simulink model "balanceLQRhostTest"  (Simulink 8.1)
settings: Solver=ode3  StartTime=0.0  StopTime=inf  RelTol=1e-3
StopFcn:
  | subplot(3,1,1);
  | plot(Data.time,Data.signals(1,1).values,'-r','LineWidth',1.5)
  | legend('Angle');
  | grid;
  | ylabel('alpha [deg]');
  | title('Pendulum');
  | subplot(3,1,2);
  | plot(Data.time,Data.signals(1,4).values,'-r','LineWidth',1.5)
  | hold on;
  | plot(Data.time,Data.signals(1,3).values,'-b','LineWidth',1.5)
  | grid;
  | legend('theta','setvalue');
  | ylabel('Arm [deg]');
  | subplot(3,1,3);
  | plot(Data.time,Data.signals(1,5).values,'-r','LineWidth',0.5)
  | legend('V');
  | grid;
  | ylabel('Voltage [V]');
libraries: aerolibconvert2 x5
settings Model: Creator=ThanhNhan  LastModifiedBy=ThanhNhan
settings DataIOCC: SignalLoggingSaveFormat=Dataset
settings OptimizationCC: ExpressionDepthLimit=128  OptimizeModelRefInitCode=on  LifeSpan=Inf
settings DebuggingCC: FcnCallInpInsideContextMsg=EnableAllAsError
settings RTWCC: SystemTargetFile=stm32f4.tlc  TemplateMakefile=ert_default_tmf  Description=STM32F4 Target  ProcessScript=stm32f4_make_rtw_hook
settings CodeAppCC: IgnoreCustomStorageClasses=off
settings STFCustomTargetCC: CodeReplacementLibrary=ANSI_C  GenerateSampleERTMain=on  ModelReferenceCompliant=off  CombineOutputUpdateFcns=on  ERTCustomFileBanners=on  SupportContinuousTime=off  SupportNonInlinedSFcns=off  MATLABClassNameForMDSCustomization=Simulink.SoftwareTarget.ERTCustomization  GRTInterface=off  SystemTargetFile=stm32f4.tlc
settings ERTTargetCC: CodeReplacementLibrary=ANSI_C  MultiwordLength=2048  GenerateSampleERTMain=on  ModelReferenceCompliant=off  ParMdlRefBuildCompliant=off  CompOptLevelCompliant=off  ConcurrentExecutionCompliant=off  ERTFirstTimeCompliant=off  ModelStepFunctionPrototypeControlCompliant=off  CPPClassGenCompliant=off  InlinedParameterPlacement=NonHierarchical  ERTCustomFileTemplate=example_file_process.tlc  ConvertIfToSwitch=off  SuppressUnreachableDefaultCases=off

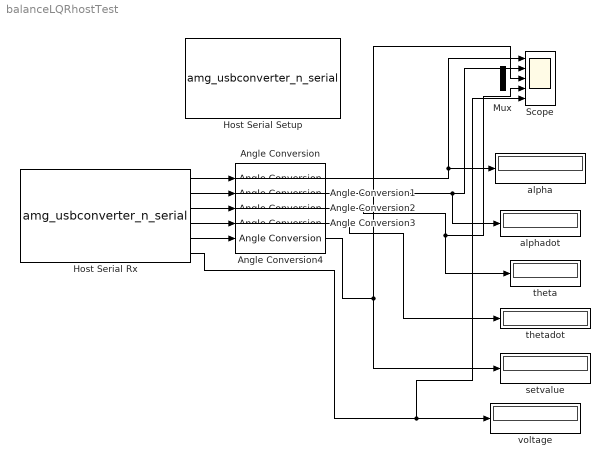
== system balanceLQRhostTest ==
  Angle Conversion{,1..4} (5 alike) : aerolibconvert2/Angle Conversion  IU=rad  OU=deg
  Host Serial Rx : S-Function  Priority=1  FunctionName=amg_usbconverter_n_serial  Parameters=configuration,port,transfer,baudrate,stopbit,inputtype,outputtype,binheaderarray,binterminatorarray,asciiheader,asciiterminator,bindatalength,packetmode,timeout,sampletime,sampletimestr,blockid  EnableBusSupport=off  mask(amg_usbconverter_n_serial){configuration=Rx, port=COM4, baudrate=115200, databits=8, parity=None, stopbit=1, flowcontrol=None, advanceoptions=off, rxbuffersize=2048, txbuffersize=2048, transfer=Blocking, timeout=5, packetmode=Binary, binheader='7E 7E', binterminator='03 03', porttype_double=6, porttype_single=0, porttype_int8=0, porttype_uint8=0, porttype_int16=0, porttype_uint16=0, porttype_int32=0, porttype_uint32=0, asciiformat='%d,%f', rx_asciiterminator=LF (0x0A - "\n"), tx_asciiterminator=LF (0x0A - "\n"), inputtype=[0], outputtype=[6  0 0 0 0 0 0], binheaderarray=[2 126  126], binterminatorarray=[2 3  3], bindatalength=48, asciiheader=['%d,%f' uint8(10)], asciiterminator=[1 10], sampletime=0.01, sampletimestr=0.01, blockid=HostSerialRx}
      mask prompts: baudrate "Baud rate (bps)"; databits "Data bits"; stopbit "Stop bit"; flowcontrol "Hardware flow control"; advanceoptions "Advance options"; rxbuffersize "Rx buffer size (bytes)"; txbuffersize "Tx buffer size (bytes)"; timeout "Wait time-out (Seconds)"; packetmode "Packet mode"; binheader "Binary header (example: '7E 7E')"; binterminator "Binary terminator (example: '03 03')"; porttype_double "Number of data port, type DOUBLE"; porttype_single "Number of data port, type SINGLE"; porttype_int8 "Number of data port, type INT8"; porttype_uint8 "Number of data port, type UINT8"; porttype_int16 "Number of data port, type INT16"; porttype_uint16 "Number of data port, type UINT16"; porttype_int32 "Number of data port, type INT32"; porttype_uint32 "Number of data port, type UINT32"; asciiformat "Ascii format"; rx_asciiterminator "End of packet"; tx_asciiterminator "End of packet"; inputtype "Input data type"; outputtype "Output data type"; binheaderarray "Binary header"; binterminatorarray "Binary terminator"; bindatalength "Binary data length"; asciiheader "Ascii header (printf format)"; asciiterminator "Ascii terminator"; sampletime "Sample time (sec)"; sampletimestr "Compiled sample time (sec) in string"
      mask init:
      | amg_usbconverter_n_serial_callback('init');
      mask Help: web(fullfile(waijungdocroot,'amg_usbconverter_n_uart.htm'), '-browser')
      mask TypeOptions configuration: Setup | Tx | Rx
      mask Callback configuration: amg_usbconverter_n_serial_callback('configuration');
      mask TypeOptions port: COM1 | COM2 | COM4
      mask Callback port: amg_usbconverter_n_serial_callback('port');
      mask Callback baudrate: amg_usbconverter_n_serial_callback('baudrate');
      mask TypeOptions databits: 8
      mask TypeOptions parity: None
      mask TypeOptions stopbit: 1 | 1.5 | 2
      mask TypeOptions flowcontrol: None | RTS | CTS | RTS/CTS
      mask Callback flowcontrol: amg_usbconverter_n_serial_callback('flowcontrol');
      mask Callback advanceoptions: amg_usbconverter_n_serial_callback('advanceoptions');
      mask TypeOptions rxbuffersize: 16 | 32 | 64 | 128 | 256 | 512 | 1024 | 2048
      mask TypeOptions txbuffersize: 16 | 32 | 64 | 128 | 256 | 512 | 1024 | 2048
      mask TypeOptions transfer: Blocking | Non-Blocking
      mask Callback transfer: amg_usbconverter_n_serial_callback('transfer');
      mask TypeOptions packetmode: Ascii | Binary
      mask Callback packetmode: amg_usbconverter_n_serial_callback('packetmode');
      mask Callback binheader: amg_usbconverter_n_serial_callback('binheader');
      mask Callback binterminator: amg_usbconverter_n_serial_callback('binterminator');
      mask Callback porttype_double: amg_usbconverter_n_serial_callback('porttype');
      mask Callback porttype_single: amg_usbconverter_n_serial_callback('porttype');
      mask Callback porttype_int8: amg_usbconverter_n_serial_callback('porttype');
      mask Callback porttype_uint8: amg_usbconverter_n_serial_callback('porttype');
      mask Callback porttype_int16: amg_usbconverter_n_serial_callback('porttype');
      mask Callback porttype_uint16: amg_usbconverter_n_serial_callback('porttype');
      mask Callback porttype_int32: amg_usbconverter_n_serial_callback('porttype');
      mask Callback porttype_uint32: amg_usbconverter_n_serial_callback('porttype');
      mask Callback asciiformat: amg_usbconverter_n_serial_callback('asciiformat');
      mask TypeOptions rx_asciiterminator: CR (0x0D - "\r") | LF (0x0A - "\n") | CRLF (0x0D 0x0A - "\r\n")
      mask Callback rx_asciiterminator: amg_usbconverter_n_serial_callback('rx_asciiterminator');
      mask TypeOptions tx_asciiterminator: CR (0x0D - "\r") | LF (0x0A - "\n") | CRLF (0x0D 0x0A - "\r\n") | None
      mask Callback tx_asciiterminator: amg_usbconverter_n_serial_callback('tx_asciiterminator');
      mask Callback sampletime: amg_usbconverter_n_serial_callback('sampletime');
      mask Callback sampletimestr: amg_usbconverter_n_serial_callback('sampletimestr');
      mask Callback blockid: amg_usbconverter_n_serial_callback('blockid');
      mask Display: text(0.05, 0.5, 'Port: COM4\nPacket: Binary\nTransfer: Blocking\nTs (sec): 0.01','ver','middle','hor','left');port_label('output', 1,'double');port_label('output', 2,'double');port_label('output', 3,'double');port_label('output', 4,'double');port_label('output', 5,'double');port_label('output', 6,'double');
  Host Serial Setup : S-Function  Priority=1  FunctionName=amg_usbconverter_n_serial  Parameters=configuration,port,transfer,baudrate,stopbit,inputtype,outputtype,binheaderarray,binterminatorarray,asciiheader,asciiterminator,bindatalength,packetmode,timeout,sampletime,sampletimestr,blockid  EnableBusSupport=off  mask(amg_usbconverter_n_serial){configuration=Setup, port=COM4, baudrate=115200, databits=8, parity=None, stopbit=1, flowcontrol=None, advanceoptions=off, rxbuffersize=2048, txbuffersize=2048, transfer=Blocking, timeout=5, packetmode=Binary, binheader='7E 7E', binterminator='03 03', porttype_double=1, porttype_single=0, porttype_int8=1, porttype_uint8=0, porttype_int16=0, porttype_uint16=0, porttype_int32=0, porttype_uint32=0, asciiformat='%d,%f', rx_asciiterminator=CRLF (0x0D 0x0A - "\r\n"), tx_asciiterminator=CR (0x0D - "\r"), inputtype=[0], outputtype=[0], binheaderarray=[2 126  126], binterminatorarray=[2 3  3], bindatalength=0, asciiheader='', asciiterminator=[0], sampletime=inf, sampletimestr=0.01, blockid=HostSerialSetup}
      mask prompts: baudrate "Baud rate (bps)"; databits "Data bits"; stopbit "Stop bit"; flowcontrol "Hardware flow control"; advanceoptions "Advance options"; rxbuffersize "Rx buffer size (bytes)"; txbuffersize "Tx buffer size (bytes)"; timeout "Wait time-out (Seconds)"; packetmode "Packet mode"; binheader "Binary header (example: '7E 7E')"; binterminator "Binary terminator (example: '03 03')"; porttype_double "Number of data port, type DOUBLE"; porttype_single "Number of data port, type SINGLE"; porttype_int8 "Number of data port, type INT8"; porttype_uint8 "Number of data port, type UINT8"; porttype_int16 "Number of data port, type INT16"; porttype_uint16 "Number of data port, type UINT16"; porttype_int32 "Number of data port, type INT32"; porttype_uint32 "Number of data port, type UINT32"; asciiformat "Ascii format"; rx_asciiterminator "End of packet"; tx_asciiterminator "End of packet"; inputtype "Input data type"; outputtype "Output data type"; binheaderarray "Binary header"; binterminatorarray "Binary terminator"; bindatalength "Binary data length"; asciiheader "Ascii header (printf format)"; asciiterminator "Ascii terminator"; sampletime "Sample time (sec)"; sampletimestr "Compiled sample time (sec) in string"
      mask init:
      | amg_usbconverter_n_serial_callback('init');
      mask Help: web(fullfile(waijungdocroot,'amg_usbconverter_n_uart.htm'), '-browser')
      mask TypeOptions configuration: Setup | Tx | Rx
      mask Callback configuration: amg_usbconverter_n_serial_callback('configuration');
      mask TypeOptions port: COM1 | COM2 | COM4
      mask Callback port: amg_usbconverter_n_serial_callback('port');
      mask Callback baudrate: amg_usbconverter_n_serial_callback('baudrate');
      mask TypeOptions databits: 8
      mask TypeOptions parity: None
      mask TypeOptions stopbit: 1 | 1.5 | 2
      mask TypeOptions flowcontrol: None | RTS | CTS | RTS/CTS
      mask Callback flowcontrol: amg_usbconverter_n_serial_callback('flowcontrol');
      mask Callback advanceoptions: amg_usbconverter_n_serial_callback('advanceoptions');
      mask TypeOptions rxbuffersize: 16 | 32 | 64 | 128 | 256 | 512 | 1024 | 2048
      mask TypeOptions txbuffersize: 16 | 32 | 64 | 128 | 256 | 512 | 1024 | 2048
      mask TypeOptions transfer: Blocking | Non-Blocking
      mask Callback transfer: amg_usbconverter_n_serial_callback('transfer');
      mask TypeOptions packetmode: Ascii | Binary
      mask Callback packetmode: amg_usbconverter_n_serial_callback('packetmode');
      mask Callback binheader: amg_usbconverter_n_serial_callback('binheader');
      mask Callback binterminator: amg_usbconverter_n_serial_callback('binterminator');
      mask Callback porttype_double: amg_usbconverter_n_serial_callback('porttype');
      mask Callback porttype_single: amg_usbconverter_n_serial_callback('porttype');
      mask Callback porttype_int8: amg_usbconverter_n_serial_callback('porttype');
      mask Callback porttype_uint8: amg_usbconverter_n_serial_callback('porttype');
      mask Callback porttype_int16: amg_usbconverter_n_serial_callback('porttype');
      mask Callback porttype_uint16: amg_usbconverter_n_serial_callback('porttype');
      mask Callback porttype_int32: amg_usbconverter_n_serial_callback('porttype');
      mask Callback porttype_uint32: amg_usbconverter_n_serial_callback('porttype');
      mask Callback asciiformat: amg_usbconverter_n_serial_callback('asciiformat');
      mask TypeOptions rx_asciiterminator: CR (0x0D - "\r") | LF (0x0A - "\n") | CRLF (0x0D 0x0A - "\r\n")
      mask Callback rx_asciiterminator: amg_usbconverter_n_serial_callback('rx_asciiterminator');
      mask TypeOptions tx_asciiterminator: CR (0x0D - "\r") | LF (0x0A - "\n") | CRLF (0x0D 0x0A - "\r\n") | None
      mask Callback tx_asciiterminator: amg_usbconverter_n_serial_callback('tx_asciiterminator');
      mask Callback sampletime: amg_usbconverter_n_serial_callback('sampletime');
      mask Callback sampletimestr: amg_usbconverter_n_serial_callback('sampletimestr');
      mask Callback blockid: amg_usbconverter_n_serial_callback('blockid');
      mask Display: text(0.5, 0.5, 'Port: COM4\nBaud (Bps): 115200\nFrame: 8-None-1','ver','middle','hor','center');
  Mux : Mux  Inputs=2
  Scope : Scope  NumInputPorts=5
      settings: YMin=0.01225~-0.2~-0.2~-0.2~-5  YMax=0.0155~0.2~1~0.2~5  SaveName=Data
  alpha : Display
  alphadot : Display
  setvalue : Display
  theta : Display
  thetadot : Display
  voltage : Display
  wires:
  Host Serial Rx/2 -> Angle Conversion1/1
  Host Serial Rx/3 -> Angle Conversion2/1
  Host Serial Rx/4 -> Angle Conversion3/1
  Host Serial Rx/5 -> Angle Conversion4/1
  Host Serial Rx/6 -> Scope/5, voltage/1
  Host Serial Rx/1 -> Angle Conversion/1
  Angle Conversion4/1 -> Scope/3, setvalue/1
  Angle Conversion/1 -> Scope/1, alpha/1
  Angle Conversion1/1 -> alphadot/1, Scope/2
  Angle Conversion2/1 -> Scope/4, theta/1
  Angle Conversion3/1 -> thetadot/1
